simulink model "redresseurrsimplecommande"  (Simulink 8.1)
settings: Solver=ode3  StartTime=0.0  StopTime=1  FixedStep=Ts  RelTol=1e-3
InitFcn:
  | Ts = 5e-5
libraries: powerlib x20, powerlib_extras x1
settings Model: Creator=LiberT  LastModifiedBy=francisvalois
settings DebuggingCC: FcnCallInpInsideContextMsg=EnableAllAsWarning
settings GRTTargetCC: CombineOutputUpdateFcns=on  GRTInterface=off

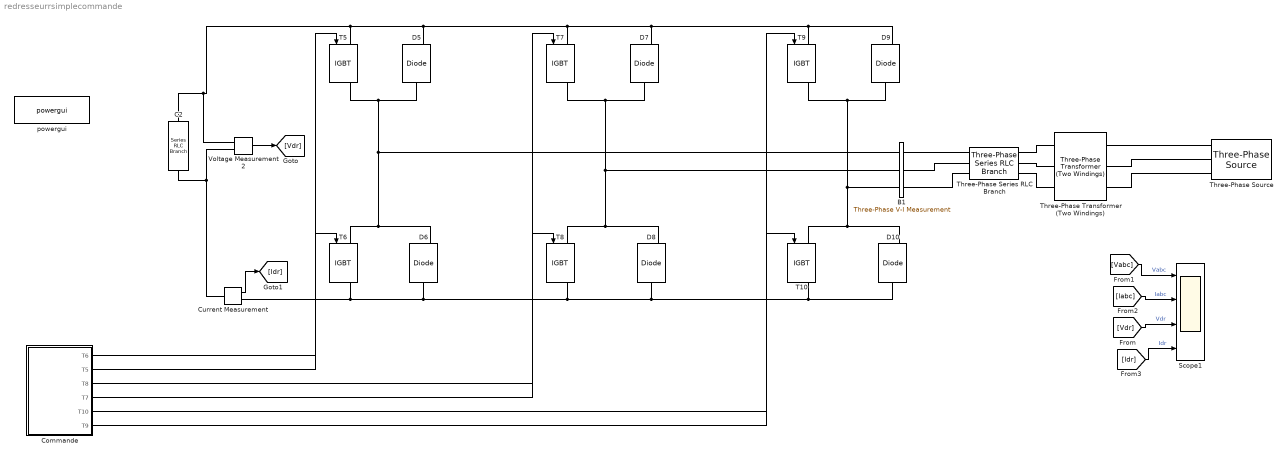
== system redresseurrsimplecommande ==
  B1 : powerlib/Measurements/Three-Phase V-I Measurement  VoltageMeasurement=phase-to-phase  SetLabelV=on  LabelV=Vabc  Vpu=off  VpuLL=off  CurrentMeasurement=yes  SetLabelI=on  LabelI=Iabc  Ipu=off  Pbase=100e6  Vbase=500e3  OutputType=Complex  PhasorSimulation=off  PSBequivalent=0
  C2 : powerlib/Elements/Series RLC Branch  LConnTagsString=__new0  RConnTagsString=__new0  BranchType=C  Resistance=0.28  Inductance=1e-3  SetiL0=off  InitialCurrent=0  Capacitance=300e-3  Setx0=off  InitialVoltage=0  Measurements=None
  Commande : Subsystem  mask{Iac=7000, Fac=50}
      mask prompts: Iac "Maximum de courant (A)"; Fac "Fréquence (Hz)"
  Current Measurement : powerlib/Measurements/Current Measurement  PhasorSimulation=off  OutputType=Complex  PSBequivalent=0
  D{5..10} (6 alike) : powerlib/Power Electronics/Diode  Ron=0.001  Lon=0  Vf=0.8  IC=0  UseSnubber=off  Rs=500  Cs=250e-9  Measurements=on
  Scope1 : Scope  NumInputPorts=4
      settings: TickLabels=on  TimeRange=0.2  YMin=-1250~-7500~1166~-5000  YMax=1250~7500~1174~5000
  T{5..10} (6 alike) : powerlib/Power Electronics/IGBT  Ron=0.001  Lon=0  Vf=1  Tf=1e-6  Tt=2e-6  IC=0  Rs=1e5  Cs=inf  Measurements=on
  Three-Phase Series RLC Branch : powerlib/Elements/Three-Phase Series RLC Branch  LConnTagsString=A|B|C  RConnTagsString=A|B|C  BranchType=RL  Resistance=0.1  Inductance=1e-8  Capacitance=1e-6  Measurements=None
  Three-Phase Transformer (Two Windings) : powerlib/Elements/Three-Phase Transformer (Two Windings)  Winding1Connection=Yg  UNITS=pu  NominalPower=[ 2500e6 , 50 ]  Winding1=[ 18e3 , 0.002 , 0.08 ]  Winding2Connection=Yg  Winding2=[ 2e3 , 0.002 , 0.08 ]  SetSaturation=off  Rm=500  Lm=500  Saturation=[ 0,0 ; 0.0024,1.2 ; 1.0,1.52 ]  Hysteresis=off  DataFile='hysteresis'  SetInitialFlux=off  InitialFluxes=[ 0.8 , -0.8 , 0.7 ]  Measurements=None  MoreParameters=off  BreakLoop=off  DataType=off  TransfoNumber=1
  Three-Phase Source : powerlib/Electrical Sources/Three-Phase Source  Voltage=18e3  PhaseAngle=0  Frequency=50  InternalConnection=Yg  SpecifyImpedance=on  Resistance=0.8929  Inductance=16.58e-3  ShortCircuitLevel=100e6  BaseVoltage=25e3  XRratio=7  BusType=swing  Pref=0  Qref=0  Qmin=-inf  Qmax=inf
  Voltage Measurement2 : powerlib/Measurements/Voltage Measurement  PhasorSimulation=off  OutputType=Complex  PSBequivalent=0
  powergui : powerlib/powergui  Priority=1  SimulationMode=Discrete  SolverType=Tustin  SampleTime=Ts  frequency=60  SPID=off  DisableSnubberDevices=off  DisableRonSwitches=off  DisableVfSwitches=off  SwTol=0  Interpol=off  DisplayEquations=off  frequencyindice=0  Pbase=100e6  ErrMax=1e-4  Iterations=50  UnitsV=kV  UnitsW=MW  FunctionMessages=off  echomessages=off  HookPort=off  EnableUseOfTLC=off  x0status=blocks  RestoreLinks=warning  ResistiveCurrentMeasurement=off  Frange=[0:2:500]  Ylog=off  Xlog=on  ShowGrid=off  save=off  variable=ZData  ZoomFFT=off  StartTime=0.0  cycles=1  DisplayStyle=1  fundamental=60  FreqAxis=off  MaxFrequency=1000  frequencyindicesteady=1  RmsSteady=1  display=off  Ts=0  methode=off
  wires:
  Voltage Measurement2/1 -> [Vdr]
  [Vdr] -> Scope1/3  "Vdr"
  Commande/6(T9) -> T9/1
  Commande/5(T10) -> T10/1
  Commande/4(T7) -> T7/1
  Commande/3(T8) -> T8/1
  [Vabc] -> Scope1/1  "Vabc"
  [Iabc] -> Scope1/2  "Iabc"
  Commande/2(T5) -> T5/1
  Commande/1(T6) -> T6/1
  Current Measurement/1 -> [Idr]
  [Idr] -> Scope1/4  "Idr"
  connections:
  Voltage Measurement2/LConn2 -- C2/RConn1 -- Current Measurement/LConn1
  T9/RConn1 -- D9/LConn1 -- T10/LConn1 -- D10/RConn1 -- B1/LConn3
  T5/LConn1 -- D5/RConn1 -- D7/RConn1 -- T9/LConn1 -- D9/RConn1 -- T7/LConn1 -- C2/LConn1 -- Voltage Measurement2/LConn1
  T8/LConn1 -- D8/RConn1 -- T7/RConn1 -- D7/LConn1 -- B1/LConn2
  T5/RConn1 -- D5/LConn1 -- T6/LConn1 -- D6/RConn1 -- B1/LConn1
  Three-Phase Source/RConn1 -- Three-Phase Transformer (Two Windings)/LConn1
  Three-Phase Series RLC Branch/RConn1 -- Three-Phase Transformer (Two Windings)/RConn1
  Three-Phase Series RLC Branch/RConn2 -- Three-Phase Transformer (Two Windings)/RConn2
  Three-Phase Series RLC Branch/RConn3 -- Three-Phase Transformer (Two Windings)/RConn3
  Three-Phase Source/RConn2 -- Three-Phase Transformer (Two Windings)/LConn2
  Three-Phase Source/RConn3 -- Three-Phase Transformer (Two Windings)/LConn3
  B1/RConn1 -- Three-Phase Series RLC Branch/LConn1
  B1/RConn2 -- Three-Phase Series RLC Branch/LConn2
  B1/RConn3 -- Three-Phase Series RLC Branch/LConn3
  T8/RConn1 -- D8/LConn1 -- T10/RConn1 -- D10/LConn1 -- D6/LConn1 -- T6/RConn1 -- Current Measurement/RConn1

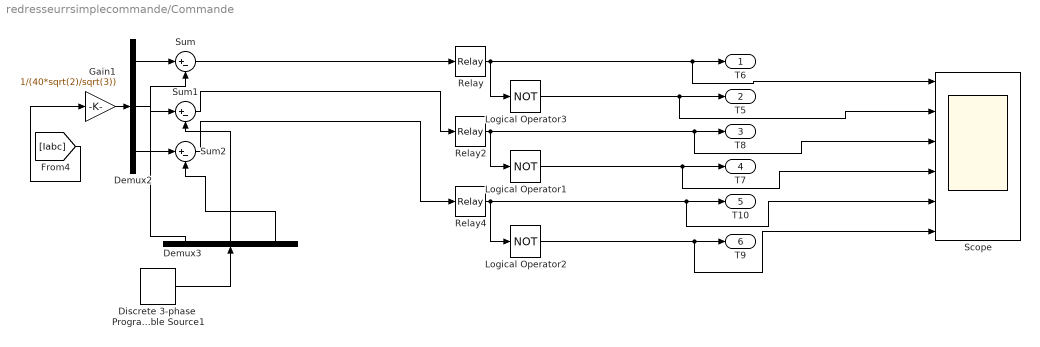
== system redresseurrsimplecommande/Commande ==
  Demux2 : Demux  Outputs=3
  Demux3 : Demux  Outputs=3
  Discrete 3-phase  Programmable Source1 : powerlib_extras/Discrete  Control Blocks/Discrete 3-phase  Programmable Source  Par_Vps=[Iac/30 90 Fac]  VariationEntity=None  VariationType=Step  VariationStep=-0.5  VariationRate=10  VariationMag=0.3  VariationFreq=2  Par_Timing_Variation=[0.1 1.2]  SinglePhase=on  Yampli=[1 0.2 1.2 1.0]  Xtime=[0 0.1 0.15 0.2]  HarmonicGeneration=off  Par_HarmoA=[3 0.2 -25 0]  Par_HarmoB=[2 0.15 35 2]  Par_Timing_Harmo="[0.05  3]"  Ts=Ts
  Gain1 : Gain  Gain=1/(40*sqrt(2)/sqrt(3))
  Logical Operator1 : Logic  Operator=NOT  AllPortsSameDT=off  OutDataTypeStr=boolean
  Logical Operator2 : Logic  Operator=NOT  AllPortsSameDT=off  OutDataTypeStr=boolean
  Logical Operator3 : Logic  Operator=NOT  AllPortsSameDT=off  OutDataTypeStr=boolean
  Relay : Relay  OnSwitchValue=0.1  OffSwitchValue=-0.1
  Relay2 : Relay  OnSwitchValue=0.1  OffSwitchValue=-0.1
  Relay4 : Relay  OnSwitchValue=0.1  OffSwitchValue=-0.1
  Scope : Scope  NumInputPorts=6
      settings: YMin=-0.1~-0.1~-0.1~-0.1~-0.1~-0.1  YMax=1.1~1.1~1.1~1.1~1.1~1.1
  Sum : Sum  Inputs=|+-
  Sum1 : Sum  Inputs=|+-
  Sum2 : Sum  Inputs=|+-
  T6 : Outport
  T5 : Outport  Port=2
  T8 : Outport  Port=3
  T7 : Outport  Port=4
  T10 : Outport  Port=5
  T9 : Outport  Port=6
  wires:
  Demux2/1 -> Sum/1
  Demux3/1 -> Sum/2
  Demux2/2 -> Sum1/1
  Demux2/3 -> Sum2/1
  Demux3/2 -> Sum1/2
  Demux3/3 -> Sum2/2
  [Iabc] -> Gain1/1
  Gain1/1 -> Demux2/1
  Discrete 3-phase  Programmable Source1/1 -> Demux3/1
  Sum/1 -> Relay/1
  Sum1/1 -> Relay2/1
  Sum2/1 -> Relay4/1
  Relay/1 -> Logical Operator3/1, Scope/1, T6/1
  Relay2/1 -> Logical Operator1/1, Scope/3, T8/1
  Logical Operator1/1 -> Scope/4, T7/1
  Relay4/1 -> Logical Operator2/1, Scope/5, T10/1
  Logical Operator2/1 -> Scope/6, T9/1
  Logical Operator3/1 -> Scope/2, T5/1
